simulink model "Prototype3C"  (R2015a)
settings: Solver=ode45  SolverMode=SingleTasking  StartTime=0.0  StopTime=17.0  RelTol=1e-3
PreLoadFcn:
  | load 'RegionInterest.mat'
undefined symbols (not defined in the file): gray, HDTV, Horn, Rec, RegionOfInterest, Schunck, strel
libraries: visionanalysis x3, visionconversions x2, visionmorphops x2, visiontransforms x2, visionsinks x2, visiontextngfix x1, visionstatistics x1, dspvision x1
settings Model: Creator=Andrew H  LastModifiedBy=Andrew
settings OptimizationCC: BlockReduction=off  BooleanDataType=off
settings DebuggingCC: SaveWithParameterizedLinksMsg=none  UnderspecifiedInitializationDetection=Classic  MergeDetectMultiDrivingBlocksExec=none  SignalResolutionControl=TryResolveAllWithWarning
settings HardwareCC: TargetUnknown=on

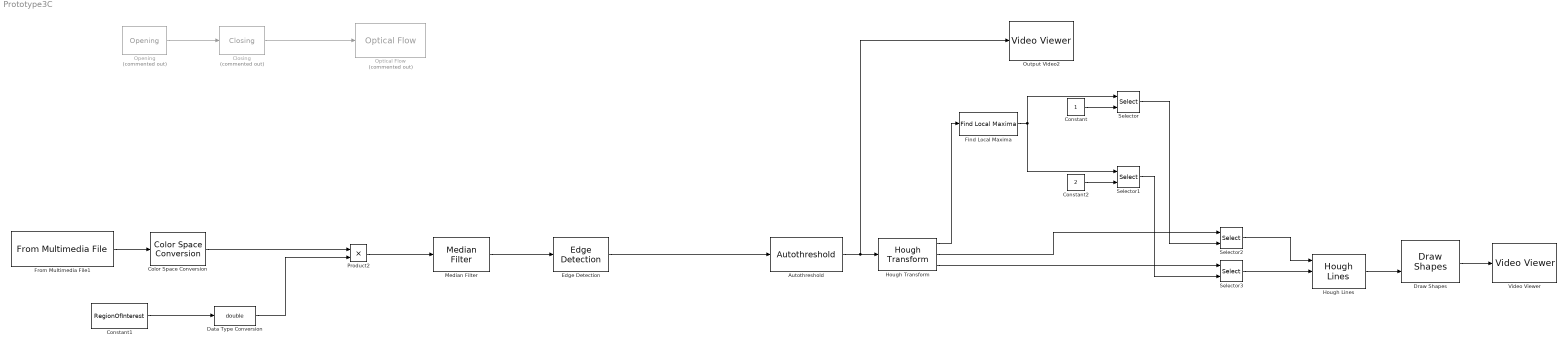
== system Prototype3C ==
  Autothreshold : visionconversions/Autothreshold  operator=>  threshOut=off  effMetricOut=off  userDefinedRange=off  umin=0  umax=255  outOfRngOpt=Warn and saturate  scaleThreshold=off  scaleFactor=1  P1Mode=Specify word length  P1WordLength=32  P1FracLength=30  P2Mode=Specify word length  P2WordLength=32  P2FracLength=22  P3Mode=Specify word length  P3WordLength=32  P3FracLength=14  P4Mode=Binary point scaling  P4WordLength=32  P4FracLength=15  Q1Mode=Specify word length  Q1WordLength=32  Q1FracLength=16  EMMode=Specify word length  EMWordLength=16  EMFracLength=14  roundingMode=Floor  overflowMode=off
  Closing : visionmorphops/Closing  Commented=on  nhoodsrc=Specify via dialog  strel=strel('line',5,45)
  Color Space Conversion : visionconversions/Color Space  Conversion  conversion=Obsolete  conversionActive=R'G'B' to intensity  wp_str=D65  rec=Rec. 709 (HDTV)  sys=1125/60/2:1  imagePorts=One multidimensional signal
  Constant : Constant
  Constant1 : Constant  Value=RegionOfInterest
  Constant2 : Constant  Value=2
  Data Type Conversion : DataTypeConversion  OutDataTypeStr=double
  Draw Shapes : visiontextngfix/Draw Shapes  shape=Lines  fill=on  lineWidth=4  fillClrSource=Specify via dialog  display=White  intensity=200  color=[255 0 0]  opacity=0.6  viewport=Entire image  antialiasing=off  inType=Obsolete  imagePorts=One multidimensional signal  prodOutputMode=Binary point scaling  prodOutputWordLength=32  prodOutputFracLength=14  memoryMode=Specify word length  memoryWordLength=16  memoryFracLength=14  roundingMode=Floor  overflowMode=off
  Edge Detection : visionanalysis/Edge Detection  method=Sobel  outputType=Binary image  userDefinedThreshold=off  thresholdSource=Input port  threshold=20  thresholdTuning=4  edgeThinning=off  threshold_canny=[0.25 0.60]  autoPercent=70  sigma=1  prodOutputMode=Binary point scaling  prodOutputWordLength=32  prodOutputFracLength=8  roundingMode=Floor  overflowMode=off
  Find Local Maxima : visionstatistics/Find Local Maxima  num_peaks=1  nhood_size=[5 7]  src_thresh=Obsolete9b  src_thresh_inuse=Specify via dialog  threshold=10  inputIsHough=on  dt_peak=uint32  isOutVarDim=on  dt_count=uint32
  From Multimedia File1 : dspvision/From Multimedia File  inputFilename=C:\Users\Andrew\Desktop\Video.mp4  loop=on  numPlays=inf  outputStreams=Video only  videoDataType=single  audioDataType=int16  inheritSampleTime=on  userDefinedSampleTime=1/30  noAudioOutput=off  isIntensityVideo=off  fourcc=RGB  colorVideoFormat=One multidimensional signal  outputEOF=off  dataOrg=Column-major  audioFrameSize=1024  computeAudioFrameSize=off  outSamplingMode=Sample based
  Hough Lines : visiontransforms/Hough Lines  sineCompMethod=Trigonometric function  thetaRes=pi/180  firstCoeffMode=Specify word length  firstCoeffWordLength=16  firstCoeffFracLength=15  prodOutputMode=Binary point scaling  prodOutputWordLength=32  prodOutputFracLength=16  roundingMode=Nearest  overflowMode=on
  Hough Transform : visiontransforms/Hough Transform  theta_res=pi/180  rho_res=1  out_theta_rho=on  outdtmode=double  firstCoeffMode=Binary point scaling  firstCoeffWordLength=16  firstCoeffFracLength=14  secondCoeffMode=Binary point scaling  secondCoeffWordLength=32  secondCoeffFracLength=16  outputMode=Binary point scaling  outputWordLength=16  outputFracLength=0  accumMode=Binary point scaling  accumWordLength=32  accumFracLength=20  prodOutputMode=Binary point scaling  prodOutputWordLength=32  prodOutputFracLength=20  memoryMode=Binary point scaling  memoryWordLength=32  memoryFracLength=16  roundingMode=Nearest  overflowMode=on
  Median Filter : visionanalysis/Median Filter  nghbood=[3 3]  outSize=Same as input port I  padType=Symmetric  padSrc=Specify via dialog  padVal=0  roundingMode=Floor  overflowMode=off
  Opening : visionmorphops/Opening  Commented=on  nhoodsrc=Specify via dialog  strel=strel('disk',5)
  Optical Flow : visionanalysis/Optical Flow  Commented=on  method=Horn-Schunck  gradMethod=Difference filter [-1 1]  which2img=Current frame and N-th frame back  N=3  outVelForm=Magnitude-squared  lambda=1  stop_criteria=When maximum number of iterations is reached  maxAllowAbsDiff=eps  maxIter=10  numInports=3  sigmaS=1.5  sigmaW=1  eigTh=0.0039  discardNormalFlow=off  outputCurrentImage=off  prodOutputMode=Binary point scaling  prodOutputWordLength=32  prodOutputFracLength=20  outputMode=Binary point scaling  outputWordLength=32  outputFracLength=20  roundingMode=Nearest  overflowMode=on
  Output Video2 : visionsinks/Video Viewer  inputType=Obsolete7b  imagePorts=One multidimensional signal  useColorMap=off  colormapValue=gray(256)  specRange=off  minInputVal=0  maxInputVal=255  FigPos=[2 1037 958 929]  AxisZoom=on  trueSizedOnce=off  OpenAtMdlStart=on  DefaultConfigurationName=vipscopes.VideoViewerScopeCfg
  Product2 : Product
  Selector : Selector  InputPortWidth=2  IndexOptions=Index vector (port)
  Selector1 : Selector  InputPortWidth=2  IndexOptions=Index vector (port)
  Selector2 : Selector  NumberOfDimensions=2  InputPortWidth=2  IndexOptions=Select all,Index vector (port)  Indices=1,1  OutputSizes=1,1
  Selector3 : Selector  NumberOfDimensions=2  InputPortWidth=2  IndexOptions=Select all,Index vector (port)  Indices=1,1  OutputSizes=1,1
  Video Viewer : visionsinks/Video Viewer  inputType=Obsolete7b  imagePorts=One multidimensional signal  useColorMap=off  colormapValue=gray(256)  specRange=off  minInputVal=0  maxInputVal=255  FigPos=[962 1037 958 929]  AxisZoom=on  trueSizedOnce=off  OpenAtMdlStart=on  DefaultConfigurationName=vipscopes.VideoViewerScopeCfg
  wires:
  Draw Shapes/1 -> Video Viewer/1
  Hough Transform/1 -> Find Local Maxima/1
  Hough Lines/1 -> Draw Shapes/2
  Find Local Maxima/1 -> Selector/1, Selector1/1
  Constant/1 -> Selector/2
  Constant2/1 -> Selector1/2
  Selector/1 -> Selector2/2
  Selector1/1 -> Selector3/2
  Hough Transform/2 -> Selector2/1
  Hough Transform/3 -> Selector3/1
  Selector3/1 -> Hough Lines/2
  Selector2/1 -> Hough Lines/1
  Opening/1 -> Closing/1
  Closing/1 -> Optical Flow/1
  Autothreshold/1 -> Output Video2/1, Hough Transform/1
  Color Space Conversion/1 -> Product2/1
  Constant1/1 -> Data Type Conversion/1
  Data Type Conversion/1 -> Product2/2
  From Multimedia File1/1 -> Color Space Conversion/1
  Median Filter/1 -> Edge Detection/1
  Product2/1 -> Median Filter/1
  Edge Detection/1 -> Autothreshold/1
